simulink model "sum1"  (R2020b)
settings: Solver=VariableStepAuto  StartTime=0.0  StopTime=10.0  RelTol=1e-3
settings Model: Creator=Shivani  LastModifiedBy=Shivani

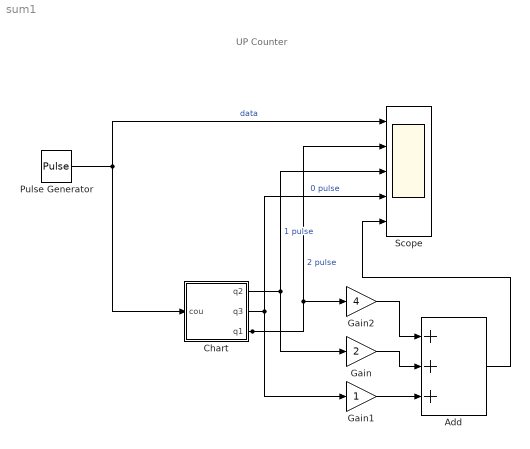
== system sum1 ==
  note: UP Counter
  Add : Sum  Inputs=+++
  Chart : Stateflow chart  TreatAsAtomicUnit=on
  Gain : Gain  Gain=2
  Gain1 : Gain
  Gain2 : Gain  Gain=4
  Pulse Generator : DiscretePulseGenerator  PulseType=Time based  Period=10  PulseWidth=50
  Scope : Scope  NumInputPorts=5
  wires:
  Chart/1(q2) -> Gain/1, Scope/3  "1 pulse"
  Add/1 -> Scope/5
  Gain1/1 -> Add/3
  Pulse Generator/1 -> Chart/1(cou), Scope/1  "data"
  Chart/2(q3) -> Scope/4, Gain1/1  "0 pulse"
  Gain/1 -> Add/2
  Gain2/1 -> Add/1
  Chart/3(q1) -> Scope/2, Gain2/1  "2 pulse"

== stateflow chart sum1/Chart ==
  state a_case5
    entry:
    q1=1;
    q2=0;
    q3=0;
  state a_case1
    entry:
    q1=0;
    q2=0;
    q3=0;
  state a000
    entry:
    q1=0;
    q2=0;
    q3=0;
  state a0004
    entry:
    q1=1;
    q2=0;
    q3=0;
  state a0001
    entry:
    q1=0;
    q2=0;
    q3=1;
  state a_case4
    entry:
    q1=0;
    q2=1;
    q3=1;
  state a_case2
    entry:
    q1=0;
    q2=0;
    q3=1;
  state a0003
    entry:
    q1=0;
    q2=1;
    q3=1;
  state a0002
    entry:
    q1=0;
    q2=1;
    q3=0;
  state a_case3
    entry:
    q1=0;
    q2=1;
    q3=0;
  (default) -> a000
  a_case5 -> a000 : [cou==1]
  a000 -> a_case1 : [cou==0]
  a0004 -> a_case5 : [cou==0]
  a_case1 -> a0001 : [cou==1]
  a_case4 -> a0004 : [cou==1]
  a0001 -> a_case2 : [cou==0]
  a0003 -> a_case4 : [cou==0]
  a_case2 -> a0002 : [cou==1]
  a_case3 -> a0003 : [cou==1]
  a0002 -> a_case3 : [cou==0]
  data: q2 output; q3 output; q1 output; cou input
